simulink model "Loadflowwithsolarbasis16kWp"  (R2023a)
settings: Solver=VariableStepAuto  StartTime=0.0  StopTime=10  RelTol=1e-3
libraries: spsThreePhaseDynamicLoadLib x20, spsThreePhaseVIMeasurementLib x18, spsThreePhaseSeriesRLCBranchLib x16, spsLoadFlowBusLib x11, spsThreePhaseParallelRLCLoadLib x10, spsRMSLib x2, spsThreePhaseTransformerTwoWindingsLib x1, spsGroundLib x1, spsThreePhaseProgrammableVoltageSourceLib x1, spspowerguiLib x1
(part 1 of 2)
settings Model: Creator=KeronDenny  LastModifiedBy=KeronDenny

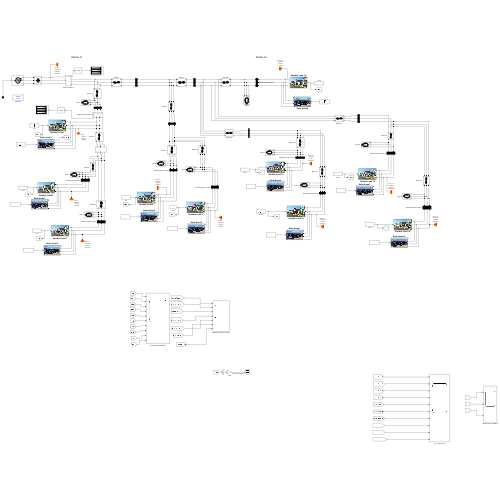
[thumbnail: Simulink's stored preview of the top-level diagram]
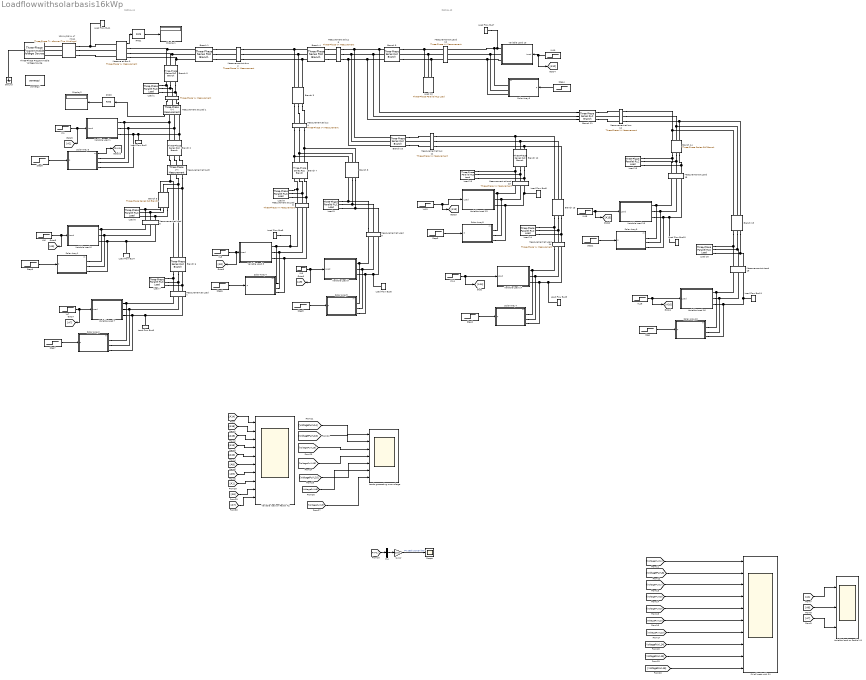
== system Loadflowwithsolarbasis16kWp ==
  note: RADIAL A1
  note: RADIAL A2
  " " : spsThreePhaseVIMeasurementLib/Three-Phase V-I Measurement  VoltageMeasurement=phase-to-ground  SetLabelV=on  LabelV=VoltagePuVL1  Vpu=on  VpuLL=off  CurrentMeasurement=no  SetLabelI=off  LabelI=Iabc  Ipu=on  Pbase=230e6  Vbase=0.230e3  OutputType=Magnitude  PhasorSimulation=on  PSBequivalent=0
  120 kV/25 kV 47 MVA1 : spsThreePhaseTransformerTwoWindingsLib/Three-Phase Transformer (Two Windings)  Winding1Connection=Yg  Winding2Connection=Yg  CoreType=Three single-phase transformers  SetSaturation=off  Hysteresis=off  DataFile='basic_model'  SetInitialFlux=off  Measurements=None  UNITS=pu  NominalPower=[230e3 50]  Winding1="[ 11e3  0.185/2/25   0.185/2 ]"  Winding2="[ 0.230e3  0.185/2/25  0.185/2]"  Rm=500  Lm=500  L0=0.5  Saturation="[ 0,0  ;  0.005,1.2  ;  1.0,1.4 ]"  InitialFluxes=[ 0.8 , -0.8 , 0.7 ]  BreakLoop=off  DiscreteSolver=Trapezoidal iterative  DataType=off  TransfoNumber=0
  Bracnh 1 : spsThreePhaseSeriesRLCBranchLib/Three-Phase Series RLC Branch  LConnTagsString=A|B|C  RConnTagsString=A|B|C  BranchType=RL  Resistance=0.216*0.240  Inductance=(0.04995*0.240)/314.159  Capacitance=1e-6  Measurements=None
  Bracnh 4 : spsThreePhaseSeriesRLCBranchLib/Three-Phase Series RLC Branch  LConnTagsString=A|B|C  RConnTagsString=A|B|C  BranchType=RL  Resistance=0.22*0.240  Inductance=(0.003*0.240)/314.159  Capacitance=1e-6  Measurements=None
  Branch 0 : spsThreePhaseSeriesRLCBranchLib/Three-Phase Series RLC Branch  LConnTagsString=A|B|C  RConnTagsString=A|B|C  BranchType=RL  Resistance=0.1824*0.240  Inductance=(0.035*0.240)/314.159  Capacitance=1e-6  Measurements=None
  Branch 10 : spsThreePhaseSeriesRLCBranchLib/Three-Phase Series RLC Branch  LConnTagsString=A|B|C  RConnTagsString=A|B|C  BranchType=RL  Resistance=0.06*0.240  Inductance=(0.004*0.240)/314.159  Capacitance=1e-6  Measurements=None
  Branch 11 : spsThreePhaseSeriesRLCBranchLib/Three-Phase Series RLC Branch  LConnTagsString=A|B|C  RConnTagsString=A|B|C  BranchType=RL  Resistance=0.032*0.240  Inductance=(0.004*0.240)/314.159  Capacitance=1e-6  Measurements=None
  Branch 12 : spsThreePhaseSeriesRLCBranchLib/Three-Phase Series RLC Branch  LConnTagsString=A|B|C  RConnTagsString=A|B|C  BranchType=RL  Resistance=0.048*0.240  Inductance=(0.003*0.240)/314.159  Capacitance=1e-6  Measurements=None
  Branch 13 : spsThreePhaseSeriesRLCBranchLib/Three-Phase Series RLC Branch  LConnTagsString=A|B|C  RConnTagsString=A|B|C  BranchType=RL  Resistance=0.042*0.240  Inductance=(0.003*0.240)/314.159  Capacitance=1e-6  Measurements=None
  Branch 14 : spsThreePhaseSeriesRLCBranchLib/Three-Phase Series RLC Branch  LConnTagsString=A|B|C  RConnTagsString=A|B|C  BranchType=RL  Resistance=0.03*0.240  Inductance=(0.002*0.240)/314.159  Capacitance=1e-6  Measurements=None
  Branch 15 : spsThreePhaseSeriesRLCBranchLib/Three-Phase Series RLC Branch  LConnTagsString=A|B|C  RConnTagsString=A|B|C  BranchType=RL  Resistance=0.042*0.240  Inductance=(0.003*0.240)/314.159  Capacitance=1e-6  Measurements=None
  Branch 2 : spsThreePhaseSeriesRLCBranchLib/Three-Phase Series RLC Branch  LConnTagsString=A|B|C  RConnTagsString=A|B|C  BranchType=RL  Resistance=0.026*0.240  Inductance=(0.003*0.240)/314.159  Capacitance=1e-6  Measurements=None
  Branch 3 : spsThreePhaseSeriesRLCBranchLib/Three-Phase Series RLC Branch  LConnTagsString=A|B|C  RConnTagsString=A|B|C  BranchType=RL  Resistance=0.06*0.240  Inductance=(0.004*0.240)/314.159  Capacitance=1e-6  Measurements=None
  Branch 5 : spsThreePhaseSeriesRLCBranchLib/Three-Phase Series RLC Branch  LConnTagsString=A|B|C  RConnTagsString=A|B|C  BranchType=RL  Resistance=0.044*0.240  Inductance=(0.003*0.240)/314.159  Capacitance=1e-6  Measurements=None
  Branch 6 : spsThreePhaseSeriesRLCBranchLib/Three-Phase Series RLC Branch  LConnTagsString=A|B|C  RConnTagsString=A|B|C  BranchType=RL  Resistance=0.023*0.240  Inductance=(0.002*0.240)/314.159  Capacitance=1e-6  Measurements=None
  Branch 7 : spsThreePhaseSeriesRLCBranchLib/Three-Phase Series RLC Branch  LConnTagsString=A|B|C  RConnTagsString=A|B|C  BranchType=RL  Resistance=0.09*0.240  Inductance=(0.006*0.240)/314.159  Capacitance=1e-6  Measurements=None
  Branch 8 : spsThreePhaseSeriesRLCBranchLib/Three-Phase Series RLC Branch  LConnTagsString=A|B|C  RConnTagsString=A|B|C  BranchType=RL  Resistance=0.072*0.240  Inductance=(0.005*0.240)/314.159  Capacitance=1e-6  Measurements=None
  Branch 9 : spsThreePhaseSeriesRLCBranchLib/Three-Phase Series RLC Branch  LConnTagsString=A|B|C  RConnTagsString=A|B|C  BranchType=RL  Resistance=0.03*0.240  Inductance=(0.002*0.240)/314.159  Capacitance=1e-6  Measurements=None
  Display1 : Display
  Display2 : Display
  Ground : spsGroundLib/Ground  LConnTagsString=a
  Load {1,6..7,13..16} (7 alike) : spsThreePhaseParallelRLCLoadLib/Three-Phase Parallel RLC Load  LConnTagsString=A|B|C  Configuration=Y (grounded)  NominalVoltage=(230)*1  Vabc=[1e3 1e3 1e3]  Vabcp=[1e3 1e3 1e3]  NominalFrequency=50  UnbalancedPower=off  ActivePower=100  InductivePower=0  CapacitivePower=2e3  Pabc=[10e3 9e3 11e3]  QLabc=[100 90 110]  QCabc=[100 90 110]  Pabcp=[10e3 9e3 11e3]  QLabcp=[100 90 110]  QCabcp=[100 90 110]  Measurements=None  LoadType=constant Z
  Load 10 : spsThreePhaseParallelRLCLoadLib/Three-Phase Parallel RLC Load  LConnTagsString=A|B|C  Configuration=Y (grounded)  NominalVoltage=(230)*1  Vabc=[1e3 1e3 1e3]  Vabcp=[1e3 1e3 1e3]  NominalFrequency=50  UnbalancedPower=off  ActivePower=100  InductivePower=0  CapacitivePower=1e3  Pabc=[10e3 9e3 11e3]  QLabc=[100 90 110]  QCabc=[100 90 110]  Pabcp=[10e3 9e3 11e3]  QLabcp=[100 90 110]  QCabcp=[100 90 110]  Measurements=None  LoadType=constant Z
  Load 8 : spsThreePhaseParallelRLCLoadLib/Three-Phase Parallel RLC Load  LConnTagsString=A|B|C  Configuration=Y (grounded)  NominalVoltage=(230)*1  Vabc=[1e3 1e3 1e3]  Vabcp=[1e3 1e3 1e3]  NominalFrequency=50  UnbalancedPower=off  ActivePower=100  InductivePower=0  CapacitivePower=1e3  Pabc=[10e3 9e3 11e3]  QLabc=[100 90 110]  QCabc=[100 90 110]  Pabcp=[10e3 9e3 11e3]  QLabcp=[100 90 110]  QCabcp=[100 90 110]  Measurements=None  LoadType=constant Z
  Load 9 : spsThreePhaseParallelRLCLoadLib/Three-Phase Parallel RLC Load  LConnTagsString=A|B|C  Configuration=Y (grounded)  NominalVoltage=(230)*1  Vabc=[1e3 1e3 1e3]  Vabcp=[1e3 1e3 1e3]  NominalFrequency=50  UnbalancedPower=off  ActivePower=100  InductivePower=0  CapacitivePower=1e3  Pabc=[10e3 9e3 11e3]  QLabc=[100 90 110]  QCabc=[100 90 110]  Pabcp=[10e3 9e3 11e3]  QLabcp=[100 90 110]  QCabcp=[100 90 110]  Measurements=None  LoadType=constant Z
  Load Flow Bus1 : spsLoadFlowBusLib/Load Flow Bus  LConnTagsString=a  Phases=single  Connectors=on one side  ID=BUS_0  Vbase=0.230e3  Vref=1  Vangle=0  VLF=0.9995  VLFb=1  VLFc=1  angleLF=3.685  angleLFb=0  angleLFc=0
  Load Flow Bus10 : spsLoadFlowBusLib/Load Flow Bus  LConnTagsString=a  Phases=single  Connectors=on one side  ID=BUS_15  Vbase=0.230e3  Vref=1  Vangle=0  VLF=1.099  VLFb=1  VLFc=1  angleLF=4.485  angleLFb=0  angleLFc=0
  Load Flow Bus11 : spsLoadFlowBusLib/Load Flow Bus  LConnTagsString=a  Phases=single  Connectors=on both sides  ID=BUS_16  Vbase=0.230e3  Vref=1  Vangle=0  VLF=1.099  VLFb=1  VLFc=1  angleLF=4.487  angleLFb=0  angleLFc=0
  Load Flow Bus2 : spsLoadFlowBusLib/Load Flow Bus  LConnTagsString=a  Phases=single  Connectors=on one side  ID=BUS_1  Vbase=0.230e3  Vref=1  Vangle=0  VLF=1.019  VLFb=1  VLFc=1  angleLF=3.896  angleLFb=0  angleLFc=0
  Load Flow Bus3 : spsLoadFlowBusLib/Load Flow Bus  LConnTagsString=a  Phases=single  Connectors=on one side  ID=BUS_7  Vbase=0.230e3  Vref=1  Vangle=0  VLF=1.021  VLFb=1  VLFc=1  angleLF=3.911  angleLFb=0  angleLFc=0
  Load Flow Bus4 : spsLoadFlowBusLib/Load Flow Bus  LConnTagsString=a  Phases=single  Connectors=on one side  ID=BUS_6  Vbase=0.230e3  Vref=1  Vangle=0  VLF=1.022  VLFb=1  VLFc=1  angleLF=3.914  angleLFb=0  angleLFc=0
  Load Flow Bus5 : spsLoadFlowBusLib/Load Flow Bus  LConnTagsString=a  Phases=single  Connectors=on one side  ID=BUS_8  Vbase=0.230e3  Vref=1  Vangle=0  VLF=1.063  VLFb=1  VLFc=1  angleLF=4.462  angleLFb=0  angleLFc=0
  Load Flow Bus6 : spsLoadFlowBusLib/Load Flow Bus  LConnTagsString=a  Phases=single  Connectors=on one side  ID=BUS_9  Vbase=0.230e3  Vref=1  Vangle=0  VLF=1.063  VLFb=1  VLFc=1  angleLF=4.46  angleLFb=0  angleLFc=0
  Load Flow Bus7 : spsLoadFlowBusLib/Load Flow Bus  LConnTagsString=a  Phases=single  Connectors=on one side  ID=BUS_10  Vbase=0.230e3  Vref=1  Vangle=0  VLF=1.097  VLFb=1  VLFc=1  angleLF=4.47  angleLFb=0  angleLFc=0
  Load Flow Bus8 : spsLoadFlowBusLib/Load Flow Bus  LConnTagsString=a  Phases=single  Connectors=on one side  ID=BUS_13  Vbase=0.230e3  Vref=1  Vangle=0  VLF=1.102  VLFb=1  VLFc=1  angleLF=4.489  angleLFb=0  angleLFc=0
  Load Flow Bus9 : spsLoadFlowBusLib/Load Flow Bus  LConnTagsString=a  Phases=single  Connectors=on one side  ID=BUS_14  Vbase=0.230e3  Vref=1  Vangle=0  VLF=1.102  VLFb=1  VLFc=1  angleLF=4.489  angleLFb=0  angleLFc=0
  Loads gnereating overvoltage : Scope  NumInputPorts=7
  Measure at Bus 0 : spsThreePhaseVIMeasurementLib/Three-Phase V-I Measurement  VoltageMeasurement=phase-to-ground  SetLabelV=off  LabelV=Vabc  Vpu=on  VpuLL=off  CurrentMeasurement=no  SetLabelI=off  LabelI=Iabc  Ipu=off  Pbase=100e6  Vbase=0.230e3  OutputType=Magnitude  PhasorSimulation=on  PSBequivalent=0
  Measurement at Laod 10 : spsThreePhaseVIMeasurementLib/Three-Phase V-I Measurement  VoltageMeasurement=phase-to-ground  SetLabelV=on  LabelV=VoltagePuVL10  Vpu=on  VpuLL=off  CurrentMeasurement=no  SetLabelI=off  LabelI=Iabc  Ipu=off  Pbase=100e6  Vbase=0.230e3  OutputType=Magnitude  PhasorSimulation=on  PSBequivalent=0
  Measurement at Laod 13 : spsThreePhaseVIMeasurementLib/Three-Phase V-I Measurement  VoltageMeasurement=phase-to-ground  SetLabelV=on  LabelV=VoltagePuVL13  Vpu=on  VpuLL=off  CurrentMeasurement=no  SetLabelI=off  LabelI=Iabc  Ipu=off  Pbase=100e6  Vbase=0.230e3  OutputType=Magnitude  PhasorSimulation=on  PSBequivalent=0
  Measurement at Load 1 : spsThreePhaseVIMeasurementLib/Three-Phase V-I Measurement  VoltageMeasurement=phase-to-ground  SetLabelV=off  LabelV=Vabc  Vpu=on  VpuLL=off  CurrentMeasurement=no  SetLabelI=off  LabelI=Iabc  Ipu=off  Pbase=100e6  Vbase=0.230e3  OutputType=Magnitude  PhasorSimulation=on  PSBequivalent=0
  Measurement at Load 14 : spsThreePhaseVIMeasurementLib/Three-Phase V-I Measurement  VoltageMeasurement=phase-to-ground  SetLabelV=on  LabelV=VoltagePuVL14  Vpu=on  VpuLL=off  CurrentMeasurement=no  SetLabelI=off  LabelI=Iabc  Ipu=off  Pbase=100e6  Vbase=0.230e3  OutputType=Magnitude  PhasorSimulation=on  PSBequivalent=0
  Measurement at Load 15 : spsThreePhaseVIMeasurementLib/Three-Phase V-I Measurement  VoltageMeasurement=phase-to-ground  SetLabelV=on  LabelV=VoltagePuVL15  Vpu=on  VpuLL=off  CurrentMeasurement=no  SetLabelI=off  LabelI=Iabc  Ipu=off  Pbase=100e6  Vbase=0.230e3  OutputType=Magnitude  PhasorSimulation=on  PSBequivalent=0
  Measurement at Load 16 : spsThreePhaseVIMeasurementLib/Three-Phase V-I Measurement  VoltageMeasurement=phase-to-ground  SetLabelV=on  LabelV=VoltagePuVL16  Vpu=on  VpuLL=off  CurrentMeasurement=no  SetLabelI=off  LabelI=Iabc  Ipu=off  Pbase=100e6  Vbase=0.230e3  OutputType=Magnitude  PhasorSimulation=on  PSBequivalent=0
  Measurement at Load 7 : spsThreePhaseVIMeasurementLib/Three-Phase V-I Measurement  VoltageMeasurement=phase-to-ground  SetLabelV=on  LabelV=VoltagePuVL7  Vpu=on  VpuLL=off  CurrentMeasurement=no  SetLabelI=off  LabelI=Iabc  Ipu=off  Pbase=100e6  Vbase=0.230e3  OutputType=Magnitude  PhasorSimulation=on  PSBequivalent=0
  Measurement at Load 8 : spsThreePhaseVIMeasurementLib/Three-Phase V-I Measurement  VoltageMeasurement=phase-to-ground  SetLabelV=on  LabelV=VoltagePuVL8  Vpu=on  VpuLL=off  CurrentMeasurement=no  SetLabelI=off  LabelI=Iabc  Ipu=off  Pbase=100e6  Vbase=0.230e3  OutputType=Magnitude  PhasorSimulation=on  PSBequivalent=0
  Measurement at Load 9 : spsThreePhaseVIMeasurementLib/Three-Phase V-I Measurement  VoltageMeasurement=phase-to-ground  SetLabelV=on  LabelV=VoltagePuVL9  Vpu=on  VpuLL=off  CurrentMeasurement=no  SetLabelI=off  LabelI=Iabc  Ipu=off  Pbase=100e6  Vbase=0.230e3  OutputType=Magnitude  PhasorSimulation=on  PSBequivalent=0
  Measurement at bus {4..5,11..12} (4 alike) : spsThreePhaseVIMeasurementLib/Three-Phase V-I Measurement  VoltageMeasurement=no  SetLabelV=off  LabelV=Vabc  Vpu=off  VpuLL=off  CurrentMeasurement=no  SetLabelI=off  LabelI=Iabc  Ipu=off  Pbase=100e6  Vbase=0.235e3  OutputType=Magnitude  PhasorSimulation=on  PSBequivalent=0
  Measurement at bus 2 : spsThreePhaseVIMeasurementLib/Three-Phase V-I Measurement  VoltageMeasurement=no  SetLabelV=off  LabelV=Vabc  Vpu=on  VpuLL=off  CurrentMeasurement=no  SetLabelI=off  LabelI=Iabc  Ipu=off  Pbase=100e6  Vbase=0.230e3  OutputType=Magnitude  PhasorSimulation=on  PSBequivalent=0
  Measurement at bus3 : spsThreePhaseVIMeasurementLib/Three-Phase V-I Measurement  VoltageMeasurement=no  SetLabelV=off  LabelV=Vabc  Vpu=off  VpuLL=on  CurrentMeasurement=no  SetLabelI=off  LabelI=Iabc  Ipu=off  Pbase=100e6  Vbase=0.230e3  OutputType=Magnitude  PhasorSimulation=on  PSBequivalent=0
  Measurement at load 6 : spsThreePhaseVIMeasurementLib/Three-Phase V-I Measurement  VoltageMeasurement=phase-to-ground  SetLabelV=on  LabelV=VoltagePuVL6  Vpu=on  VpuLL=off  CurrentMeasurement=no  SetLabelI=off  LabelI=Iabc  Ipu=off  Pbase=100e6  Vbase=0.230e3  OutputType=Magnitude  PhasorSimulation=on  PSBequivalent=0
  Mux : Mux  Inputs=1
  PU of loads with PV : Scope  NumInputPorts=10
  RMS1 : spsRMSLib/RMS  TrueRMS=on  Freq=50  RMSInit=0  Ts=0
  RMS3 : spsRMSLib/RMS  TrueRMS=on  Freq=50  RMSInit=0  Ts=0
  Scope : Scope
  Solar Array1 : Subsystem  mask(Grid-Connected PV Array (PQ Model)){Vn=230, Fn=50, P0=2000}
      mask prompts: Vn "Nominal L-L Voltage [Vrms]"; Fn "Nominal Frequency [Hz]"; P0 "Initial Power [W]"
      mask help:
      | This block models a grid-connected solar array using the Three-Phase Dynamic Load block. This is a system-level model that does not contain any power electronics, but is useful for load flow, phasor, and hybrid phasor-EMT simulations. The input to this block is the power output of the grid connected PV array, not irradiance.
      |
      | For more detailed PV models, consider the PV Array block in the Renewables library. Consider using this PQ Model to perform load flow studies and switch to a more detailed model when full EMT studies are required.
      |
      | Note: The array power must be specified for use for Load Flow analysis.
      mask init:
      | % P0 = Irr0*TotalArea*Efficiency/100;
      | P0 = -P0;
      mask Display:
      | image(imread('PV_Farm.jpg'))
      | color('white')
      | port_label('input',1,'P')
      | port_label('output',1,'m')
      | port_label('Rconn',1,'A')
      | port_label('Rconn',2,'B')
      | port_label('Rconn',3,'C')
  Solar Array10 : Subsystem  mask(Grid-Connected PV Array (PQ Model)){Vn=230, Fn=50, P0=2000}
      mask prompts: Vn "Nominal L-L Voltage [Vrms]"; Fn "Nominal Frequency [Hz]"; P0 "Initial Power [W]"
      mask help:
      | This block models a grid-connected solar array using the Three-Phase Dynamic Load block. This is a system-level model that does not contain any power electronics, but is useful for load flow, phasor, and hybrid phasor-EMT simulations. The input to this block is the power output of the grid connected PV array, not irradiance.
      |
      | For more detailed PV models, consider the PV Array block in the Renewables library. Consider using this PQ Model to perform load flow studies and switch to a more detailed model when full EMT studies are required.
      |
      | Note: The array power must be specified for use for Load Flow analysis.
      mask init:
      | % P0 = Irr0*TotalArea*Efficiency/100;
      | P0 = -P0;
      mask Display:
      | image(imread('PV_Farm.jpg'))
      | color('white')
      | port_label('input',1,'P')
      | port_label('output',1,'m')
      | port_label('Rconn',1,'A')
      | port_label('Rconn',2,'B')
      | port_label('Rconn',3,'C')
  Solar Array2 : Subsystem  mask(Grid-Connected PV Array (PQ Model)){Vn=230, Fn=50, P0=2000}
      mask prompts: Vn "Nominal L-L Voltage [Vrms]"; Fn "Nominal Frequency [Hz]"; P0 "Initial Power [W]"
      mask help:
      | This block models a grid-connected solar array using the Three-Phase Dynamic Load block. This is a system-level model that does not contain any power electronics, but is useful for load flow, phasor, and hybrid phasor-EMT simulations. The input to this block is the power output of the grid connected PV array, not irradiance.
      |
      | For more detailed PV models, consider the PV Array block in the Renewables library. Consider using this PQ Model to perform load flow studies and switch to a more detailed model when full EMT studies are required.
      |
      | Note: The array power must be specified for use for Load Flow analysis.
      mask init:
      | % P0 = Irr0*TotalArea*Efficiency/100;
      | P0 = -P0;
      mask Display:
      | image(imread('PV_Farm.jpg'))
      | color('white')
      | port_label('input',1,'P')
      | port_label('output',1,'m')
      | port_label('Rconn',1,'A')
      | port_label('Rconn',2,'B')
      | port_label('Rconn',3,'C')
  Solar Array3 : Subsystem  mask(Grid-Connected PV Array (PQ Model)){Vn=230, Fn=50, P0=2000}
      mask prompts: Vn "Nominal L-L Voltage [Vrms]"; Fn "Nominal Frequency [Hz]"; P0 "Initial Power [W]"
      mask help:
      | This block models a grid-connected solar array using the Three-Phase Dynamic Load block. This is a system-level model that does not contain any power electronics, but is useful for load flow, phasor, and hybrid phasor-EMT simulations. The input to this block is the power output of the grid connected PV array, not irradiance.
      |
      | For more detailed PV models, consider the PV Array block in the Renewables library. Consider using this PQ Model to perform load flow studies and switch to a more detailed model when full EMT studies are required.
      |
      | Note: The array power must be specified for use for Load Flow analysis.
      mask init:
      | % P0 = Irr0*TotalArea*Efficiency/100;
      | P0 = -P0;
      mask Display:
      | image(imread('PV_Farm.jpg'))
      | color('white')
      | port_label('input',1,'P')
      | port_label('output',1,'m')
      | port_label('Rconn',1,'A')
      | port_label('Rconn',2,'B')
      | port_label('Rconn',3,'C')
  Solar Array4 : Subsystem  mask(Grid-Connected PV Array (PQ Model)){Vn=230, Fn=50, P0=2000}
      mask prompts: Vn "Nominal L-L Voltage [Vrms]"; Fn "Nominal Frequency [Hz]"; P0 "Initial Power [W]"
      mask help:
      | This block models a grid-connected solar array using the Three-Phase Dynamic Load block. This is a system-level model that does not contain any power electronics, but is useful for load flow, phasor, and hybrid phasor-EMT simulations. The input to this block is the power output of the grid connected PV array, not irradiance.
      |
      | For more detailed PV models, consider the PV Array block in the Renewables library. Consider using this PQ Model to perform load flow studies and switch to a more detailed model when full EMT studies are required.
      |
      | Note: The array power must be specified for use for Load Flow analysis.
      mask init:
      | % P0 = Irr0*TotalArea*Efficiency/100;
      | P0 = -P0;
      mask Display:
      | image(imread('PV_Farm.jpg'))
      | color('white')
      | port_label('input',1,'P')
      | port_label('output',1,'m')
      | port_label('Rconn',1,'A')
      | port_label('Rconn',2,'B')
      | port_label('Rconn',3,'C')
  Solar Array5 : Subsystem  mask(Grid-Connected PV Array (PQ Model)){Vn=230, Fn=50, P0=2000}
      mask prompts: Vn "Nominal L-L Voltage [Vrms]"; Fn "Nominal Frequency [Hz]"; P0 "Initial Power [W]"
      mask help:
      | This block models a grid-connected solar array using the Three-Phase Dynamic Load block. This is a system-level model that does not contain any power electronics, but is useful for load flow, phasor, and hybrid phasor-EMT simulations. The input to this block is the power output of the grid connected PV array, not irradiance.
      |
      | For more detailed PV models, consider the PV Array block in the Renewables library. Consider using this PQ Model to perform load flow studies and switch to a more detailed model when full EMT studies are required.
      |
      | Note: The array power must be specified for use for Load Flow analysis.
      mask init:
      | % P0 = Irr0*TotalArea*Efficiency/100;
      | P0 = -P0;
      mask Display:
      | image(imread('PV_Farm.jpg'))
      | color('white')
      | port_label('input',1,'P')
      | port_label('output',1,'m')
      | port_label('Rconn',1,'A')
      | port_label('Rconn',2,'B')
      | port_label('Rconn',3,'C')
  Solar Array6 : Subsystem  mask(Grid-Connected PV Array (PQ Model)){Vn=230, Fn=50, P0=2000}
      mask prompts: Vn "Nominal L-L Voltage [Vrms]"; Fn "Nominal Frequency [Hz]"; P0 "Initial Power [W]"
      mask help:
      | This block models a grid-connected solar array using the Three-Phase Dynamic Load block. This is a system-level model that does not contain any power electronics, but is useful for load flow, phasor, and hybrid phasor-EMT simulations. The input to this block is the power output of the grid connected PV array, not irradiance.
      |
      | For more detailed PV models, consider the PV Array block in the Renewables library. Consider using this PQ Model to perform load flow studies and switch to a more detailed model when full EMT studies are required.
      |
      | Note: The array power must be specified for use for Load Flow analysis.
      mask init:
      | % P0 = Irr0*TotalArea*Efficiency/100;
      | P0 = -P0;
      mask Display:
      | image(imread('PV_Farm.jpg'))
      | color('white')
      | port_label('input',1,'P')
      | port_label('output',1,'m')
      | port_label('Rconn',1,'A')
      | port_label('Rconn',2,'B')
      | port_label('Rconn',3,'C')
  Solar Array7 : Subsystem  mask(Grid-Connected PV Array (PQ Model)){Vn=230, Fn=50, P0=2000}
      mask prompts: Vn "Nominal L-L Voltage [Vrms]"; Fn "Nominal Frequency [Hz]"; P0 "Initial Power [W]"
      mask help:
      | This block models a grid-connected solar array using the Three-Phase Dynamic Load block. This is a system-level model that does not contain any power electronics, but is useful for load flow, phasor, and hybrid phasor-EMT simulations. The input to this block is the power output of the grid connected PV array, not irradiance.
      |
      | For more detailed PV models, consider the PV Array block in the Renewables library. Consider using this PQ Model to perform load flow studies and switch to a more detailed model when full EMT studies are required.
      |
      | Note: The array power must be specified for use for Load Flow analysis.
      mask init:
      | % P0 = Irr0*TotalArea*Efficiency/100;
      | P0 = -P0;
      mask Display:
      | image(imread('PV_Farm.jpg'))
      | color('white')
      | port_label('input',1,'P')
      | port_label('output',1,'m')
      | port_label('Rconn',1,'A')
      | port_label('Rconn',2,'B')
      | port_label('Rconn',3,'C')
  Solar Array8 : Subsystem  mask(Grid-Connected PV Array (PQ Model)){Vn=230, Fn=50, P0=2000}
      mask prompts: Vn "Nominal L-L Voltage [Vrms]"; Fn "Nominal Frequency [Hz]"; P0 "Initial Power [W]"
      mask help:
      | This block models a grid-connected solar array using the Three-Phase Dynamic Load block. This is a system-level model that does not contain any power electronics, but is useful for load flow, phasor, and hybrid phasor-EMT simulations. The input to this block is the power output of the grid connected PV array, not irradiance.
      |
      | For more detailed PV models, consider the PV Array block in the Renewables library. Consider using this PQ Model to perform load flow studies and switch to a more detailed model when full EMT studies are required.
      |
      | Note: The array power must be specified for use for Load Flow analysis.
      mask init:
      | % P0 = Irr0*TotalArea*Efficiency/100;
      | P0 = -P0;
      mask Display:
      | image(imread('PV_Farm.jpg'))
      | color('white')
      | port_label('input',1,'P')
      | port_label('output',1,'m')
      | port_label('Rconn',1,'A')
      | port_label('Rconn',2,'B')
      | port_label('Rconn',3,'C')
  Solar Array9 : Subsystem  mask(Grid-Connected PV Array (PQ Model)){Vn=230, Fn=50, P0=2000}
      mask prompts: Vn "Nominal L-L Voltage [Vrms]"; Fn "Nominal Frequency [Hz]"; P0 "Initial Power [W]"
      mask help:
      | This block models a grid-connected solar array using the Three-Phase Dynamic Load block. This is a system-level model that does not contain any power electronics, but is useful for load flow, phasor, and hybrid phasor-EMT simulations. The input to this block is the power output of the grid connected PV array, not irradiance.
      |
      | For more detailed PV models, consider the PV Array block in the Renewables library. Consider using this PQ Model to perform load flow studies and switch to a more detailed model when full EMT studies are required.
      |
      | Note: The array power must be specified for use for Load Flow analysis.
      mask init:
      | % P0 = Irr0*TotalArea*Efficiency/100;
      | P0 = -P0;
      mask Display:
      | image(imread('PV_Farm.jpg'))
      | color('white')
      | port_label('input',1,'P')
      | port_label('output',1,'m')
      | port_label('Rconn',1,'A')
      | port_label('Rconn',2,'B')
      | port_label('Rconn',3,'C')
  Step{,1..9} (10 alike) : Step  Time=5  Before=2000  After=16300  SampleTime=0
  Three-Phase Programmable Voltage Source : spsThreePhaseProgrammableVoltageSourceLib/Three-Phase Programmable Voltage Source  PositiveSequence=[(11000)*1 0 50]  VariationEntity=None  VariationType=Modulation  VariationTypeAlt=Step  VariationStep=0.5  VariationRate=0.1  VariationMagnitude=0.05  VariationFrequency=1  VariationTiming=[0.1 1.2]  VariationPhaseA=off  Amplitudes=[1 0.8 1.2 1.0]  TimeValues=[0 0.1 0.15 0.2]  HarmonicGeneration=off  HarmonicA=[3 0.2 -25 0]  HarmonicB=[2 0.15 35 2]  Timing="[0.05  3]"  BusType=swing  Pref=0  Qref=0  Qmin=-Inf  Qmax=Inf
  VL1 : Step  Time=1.5  Before=1e2  After=6.119e3  SampleTime=0
  VL10 : Step  Time=0.2  Before=1e2  After=5.191e3  SampleTime=0
  VL13 : Step  Time=0.6  Before=2e2  After=7.979e3  SampleTime=0
  VL14 : Step  Before=9e2  After=5.457e3  SampleTime=0
  VL15 : Step  Time=0.1  Before=6e2  After=5.473e3  SampleTime=0
  VL16 : Step  Time=0.5  Before=10  After=5.191e3  SampleTime=0
  VL6 : Step  Time=0.9  Before=4e2  After=2.018e3  SampleTime=0
  VL7 : Step  Time=0.3  Before=8e2  After=5.178e3  SampleTime=0
  VL8 : Step  Time=0.5  Before=1e2  After=6.662e3  SampleTime=0
  VL9 : Step  Time=1.5  Before=1e2  After=3.414e3  SampleTime=0
  Variable Load 1 : Subsystem  mask(Variable Load (PQ Model)){Vn=230, Fn=50, PF=1, Load0=1e2}
      mask prompts: Vn "Nominal L-L Voltage [Vrms]"; Fn "Nominal Frequency [Hz]"; PF "Power Factor [0 to 1]"; Load0 "Initial Load [W]"
      mask help:
      | The Variable Load block is a lumped approximation for a distribution feeder. For non-unity power factor loads, the input (active power) is scaled accordingly to generate a desired load.
      |
      | Note: The initial input load must be specified for use for Load Flow analysis.
      mask init:
      | P0 = Load0;
      | Q0 = Load0*sqrt(1/PF-1);
      mask Display:
      | image(imread('Residential.jpg'))
      | color('white')
      | port_label('input',1,'Load')
      | port_label('Rconn',1,'A')
      | port_label('Rconn',2,'B')
      | port_label('Rconn',3,'C')
  Variable Load 10 : Subsystem  mask(Variable Load (PQ Model)){Vn=230, Fn=50, PF=1, Load0=1e2}
      mask prompts: Vn "Nominal L-L Voltage [Vrms]"; Fn "Nominal Frequency [Hz]"; PF "Power Factor [0 to 1]"; Load0 "Initial Load [W]"
      mask help:
      | The Variable Load block is a lumped approximation for a distribution feeder. For non-unity power factor loads, the input (active power) is scaled accordingly to generate a desired load.
      |
      | Note: The initial input load must be specified for use for Load Flow analysis.
      mask init:
      | P0 = Load0;
      | Q0 = Load0*sqrt(1/PF-1);
      mask Display:
      | image(imread('Residential.jpg'))
      | color('white')
      | port_label('input',1,'Load')
      | port_label('Rconn',1,'A')
      | port_label('Rconn',2,'B')
      | port_label('Rconn',3,'C')
  Variable Load 13 : Subsystem  mask(Variable Load (PQ Model)){Vn=230, Fn=50, PF=1, Load0=1e2}
      mask prompts: Vn "Nominal L-L Voltage [Vrms]"; Fn "Nominal Frequency [Hz]"; PF "Power Factor [0 to 1]"; Load0 "Initial Load [W]"
      mask help:
      | The Variable Load block is a lumped approximation for a distribution feeder. For non-unity power factor loads, the input (active power) is scaled accordingly to generate a desired load.
      |
      | Note: The initial input load must be specified for use for Load Flow analysis.
      mask init:
      | P0 = Load0;
      | Q0 = Load0*sqrt(1/PF-1);
      mask Display:
      | image(imread('Residential.jpg'))
      | color('white')
      | port_label('input',1,'Load')
      | port_label('Rconn',1,'A')
      | port_label('Rconn',2,'B')
      | port_label('Rconn',3,'C')
  Variable Load 14 : Subsystem  mask(Variable Load (PQ Model)){Vn=230, Fn=50, PF=1, Load0=1e2}
      mask prompts: Vn "Nominal L-L Voltage [Vrms]"; Fn "Nominal Frequency [Hz]"; PF "Power Factor [0 to 1]"; Load0 "Initial Load [W]"
      mask help:
      | The Variable Load block is a lumped approximation for a distribution feeder. For non-unity power factor loads, the input (active power) is scaled accordingly to generate a desired load.
      |
      | Note: The initial input load must be specified for use for Load Flow analysis.
      mask init:
      | P0 = Load0;
      | Q0 = Load0*sqrt(1/PF-1);
      mask Display:
      | image(imread('Residential.jpg'))
      | color('white')
      | port_label('input',1,'Load')
      | port_label('Rconn',1,'A')
      | port_label('Rconn',2,'B')
      | port_label('Rconn',3,'C')
  Variable Load 15 : Subsystem  mask(Variable Load (PQ Model)){Vn=230, Fn=50, PF=1, Load0=1e2}
      mask prompts: Vn "Nominal L-L Voltage [Vrms]"; Fn "Nominal Frequency [Hz]"; PF "Power Factor [0 to 1]"; Load0 "Initial Load [W]"
      mask help:
      | The Variable Load block is a lumped approximation for a distribution feeder. For non-unity power factor loads, the input (active power) is scaled accordingly to generate a desired load.
      |
      | Note: The initial input load must be specified for use for Load Flow analysis.
      mask init:
      | P0 = Load0;
      | Q0 = Load0*sqrt(1/PF-1);
      mask Display:
      | image(imread('Residential.jpg'))
      | color('white')
      | port_label('input',1,'Load')
      | port_label('Rconn',1,'A')
      | port_label('Rconn',2,'B')
      | port_label('Rconn',3,'C')
  Variable Load 16 : Subsystem  mask(Variable Load (PQ Model)){Vn=230, Fn=50, PF=1, Load0=1e2}
      mask prompts: Vn "Nominal L-L Voltage [Vrms]"; Fn "Nominal Frequency [Hz]"; PF "Power Factor [0 to 1]"; Load0 "Initial Load [W]"
      mask help:
      | The Variable Load block is a lumped approximation for a distribution feeder. For non-unity power factor loads, the input (active power) is scaled accordingly to generate a desired load.
      |
      | Note: The initial input load must be specified for use for Load Flow analysis.
      mask init:
      | P0 = Load0;
      | Q0 = Load0*sqrt(1/PF-1);
      mask Display:
      | image(imread('Residential.jpg'))
      | color('white')
      | port_label('input',1,'Load')
      | port_label('Rconn',1,'A')
      | port_label('Rconn',2,'B')
      | port_label('Rconn',3,'C')
  Variable Load 6 : Subsystem  mask(Variable Load (PQ Model)){Vn=230, Fn=50, PF=1, Load0=7500}
      mask prompts: Vn "Nominal L-L Voltage [Vrms]"; Fn "Nominal Frequency [Hz]"; PF "Power Factor [0 to 1]"; Load0 "Initial Load [W]"
      mask help:
      | The Variable Load block is a lumped approximation for a distribution feeder. For non-unity power factor loads, the input (active power) is scaled accordingly to generate a desired load.
      |
      | Note: The initial input load must be specified for use for Load Flow analysis.
      mask init:
      | P0 = Load0;
      | Q0 = Load0*sqrt(1/PF-1);
      mask Display:
      | image(imread('Residential.jpg'))
      | color('white')
      | port_label('input',1,'Load')
      | port_label('Rconn',1,'A')
      | port_label('Rconn',2,'B')
      | port_label('Rconn',3,'C')
  Variable Load 7 : Subsystem  mask(Variable Load (PQ Model)){Vn=230, Fn=50, PF=1, Load0=1e2}
      mask prompts: Vn "Nominal L-L Voltage [Vrms]"; Fn "Nominal Frequency [Hz]"; PF "Power Factor [0 to 1]"; Load0 "Initial Load [W]"
      mask help:
      | The Variable Load block is a lumped approximation for a distribution feeder. For non-unity power factor loads, the input (active power) is scaled accordingly to generate a desired load.
      |
      | Note: The initial input load must be specified for use for Load Flow analysis.
      mask init:
      | P0 = Load0;
      | Q0 = Load0*sqrt(1/PF-1);
      mask Display:
      | image(imread('Residential.jpg'))
      | color('white')
      | port_label('input',1,'Load')
      | port_label('Rconn',1,'A')
      | port_label('Rconn',2,'B')
      | port_label('Rconn',3,'C')
  Variable Load 8 : Subsystem  mask(Variable Load (PQ Model)){Vn=230, Fn=50, PF=1, Load0=1e2}
      mask prompts: Vn "Nominal L-L Voltage [Vrms]"; Fn "Nominal Frequency [Hz]"; PF "Power Factor [0 to 1]"; Load0 "Initial Load [W]"
      mask help:
      | The Variable Load block is a lumped approximation for a distribution feeder. For non-unity power factor loads, the input (active power) is scaled accordingly to generate a desired load.
      |
      | Note: The initial input load must be specified for use for Load Flow analysis.
      mask init:
      | P0 = Load0;
      | Q0 = Load0*sqrt(1/PF-1);
      mask Display:
      | image(imread('Residential.jpg'))
      | color('white')
      | port_label('input',1,'Load')
      | port_label('Rconn',1,'A')
      | port_label('Rconn',2,'B')
      | port_label('Rconn',3,'C')
  Variable Load 9 : Subsystem  mask(Variable Load (PQ Model)){Vn=230, Fn=50, PF=1, Load0=1e2}
      mask prompts: Vn "Nominal L-L Voltage [Vrms]"; Fn "Nominal Frequency [Hz]"; PF "Power Factor [0 to 1]"; Load0 "Initial Load [W]"
      mask help:
      | The Variable Load block is a lumped approximation for a distribution feeder. For non-unity power factor loads, the input (active power) is scaled accordingly to generate a desired load.
      |
      | Note: The initial input load must be specified for use for Load Flow analysis.
      mask init:
      | P0 = Load0;
      | Q0 = Load0*sqrt(1/PF-1);
      mask Display:
      | image(imread('Residential.jpg'))
      | color('white')
      | port_label('input',1,'Load')
      | port_label('Rconn',1,'A')
      | port_label('Rconn',2,'B')
      | port_label('Rconn',3,'C')
  Variable load on Radial A1 : Scope  NumInputPorts=3
  Variable load on Radial A2 : Scope  NumInputPorts=10
  powergui : spspowerguiLib/powergui  Priority=1  SimulationMode=Phasor  SampleTime=50e-6  frequency=50  Iterations=50  frequencyindice=50  Pbase=100e3  ErrMax=1e-4  UnitsV=kV  UnitsW=MW  buscounter=0  FunctionMessages=off  echomessages=off  EnableUseOfTLC=off  CurrentSourceSwitches=off  DisableSnubberDevices=off  DisableRonSwitches=off  DisableVfSwitches=off  DisplayEquations=off  AutomaticDiscreteSolvers=off  SolverType=Tustin/Backward Euler (TBE)  Interpol=off  ExternalGateDelay=off  methode=off  Ts=100  x0status=blocks  SPID=on  SwTol=0  HookPort=off  NonlinearTolerance=1e-4  nMaxIteration=100  ContinueOnMaxIteration=off  RestoreLinks=warning  ResistiveCurrentMeasurement=off  Frange=[0:2:500]  Ylog=off  Xlog=on  ShowGrid=off  save=off  variable=ZData  structure=0  ZoomFFT=off  StartTime=0.0  cycles=1  DisplayStyle=1  fundamental=60  FreqAxis=off  MaxFrequency=1000  frequencyindicesteady=1  RmsSteady=1  display=off
  to kW : Gain  Gain=1e-3
  wires:
  Measure at Bus 0/1 -> RMS1/1
  RMS1/1 -> Display1/1
  Measurement at Load 1/1 -> RMS3/1
  RMS3/1 -> Display2/1
  VL6/1 -> [A6], Variable Load 6/1(Load)
  VL1/1 -> [A1], Variable Load 1/1(Load)
  VL7/1 -> [A7], Variable Load 7/1(Load)
  VL8/1 -> [A8], Variable Load 8/1(Load)
  VL9/1 -> [A9], Variable Load 9/1(Load)
  VL15/1 -> Variable Load 15/1(Load), [A15]
  VL16/1 -> Variable Load 16/1(Load), [A16]
  VL14/1 -> Variable Load 14/1(Load), [A14]
  [A14] -> Variable load on Radial A2/1
  [A16] -> Variable load on Radial A2/2
  [A15] -> Variable load on Radial A2/3
  VL13/1 -> Variable Load 13/1(Load), [A13]
  [A13] -> Variable load on Radial A2/4
  VL10/1 -> [A10], Variable Load 10/1(Load)
  [A10] -> Variable load on Radial A2/5
  [A9] -> Variable load on Radial A2/7
  [A8] -> Variable load on Radial A2/6
  [A1] -> Variable load on Radial A1/1
  [A6] -> Variable load on Radial A1/2
  [A7] -> Variable load on Radial A1/3
  Solar Array3/1(m) -> [PVM1]
  Mux/1 -> to kW/1
  to kW/1 -> Scope/1  "PV peak power (kW)"
  [PVM1] -> Mux/1
  Step4/1 -> Solar Array6/1(P)
  Step/1 -> Solar Array10/1(P)
  Step1/1 -> Solar Array9/1(P)
  [VoltagePuVL6] -> PU of loads with PV/2
  [VoltagePuVL1] -> PU of loads with PV/1
  [VoltagePuVL7] -> PU of loads with PV/3
  [VoltagePuVL8] -> PU of loads with PV/4
  [VoltagePuVL9] -> PU of loads with PV/5
  [VoltagePuVL10] -> PU of loads with PV/6
  [VoltagePuVL13] -> PU of loads with PV/7
  [VoltagePuVL14] -> PU of loads with PV/8
  [VoltagePuVL15] -> PU of loads with PV/9
  [VoltagePuVL16] -> PU of loads with PV/10
  [VoltagePuVL14] -> Loads gnereating overvoltage/1
  [VoltagePuVL13] -> Loads gnereating overvoltage/2
  [VoltagePuVL16] -> Loads gnereating overvoltage/3
  [VoltagePuVL15] -> Loads gnereating overvoltage/4
  Step2/1 -> Solar Array7/1(P)
  Step3/1 -> Solar Array8/1(P)
  Step5/1 -> Solar Array5/1(P)
  Step6/1 -> Solar Array4/1(P)
  Step7/1 -> Solar Array2/1(P)
  Step9/1 -> Solar Array1/1(P)
  [VoltagePuVL10] -> Loads gnereating overvoltage/5
  Step8/1 -> Solar Array3/1(P)
  [VoltagePuVL8] -> Loads gnereating overvoltage/6
  [VoltagePuVL9] -> Loads gnereating overvoltage/7
  [A1] -> Variable load on Radial A2/8
  [A6] -> Variable load on Radial A2/9
  [A7] -> Variable load on Radial A2/10
  connections:
  Branch 0/RConn3 -- Load 1/LConn3 -- " "/LConn3
  Branch 0/RConn2 -- Load 1/LConn2 -- " "/LConn2
  Branch 0/RConn1 -- " "/LConn1 -- Load 1/LConn1
  Measurement at Load 1/LConn1 -- " "/RConn1
  Measurement at Load 1/LConn2 -- " "/RConn2
  Measurement at Load 1/LConn3 -- " "/RConn3
  Three-Phase Programmable Voltage Source/LConn1 -- Ground/LConn1
  Branch 2/LConn1 -- Solar Array3/RConn1 -- Variable Load 1/RConn1 -- Measurement at Load 1/RConn1
  Branch 2/LConn2 -- Solar Array3/RConn2 -- Variable Load 1/RConn2 -- Measurement at Load 1/RConn2
  Measurement at Load 1/RConn3 -- Solar Array3/RConn3 -- Variable Load 1/RConn3 -- Load Flow Bus2/LConn1 -- Branch 2/LConn3
  Measure at Bus 0/RConn1 -- Bracnh 1/LConn1 -- Branch 0/LConn1
  Measure at Bus 0/RConn2 -- Bracnh 1/LConn2 -- Branch 0/LConn2
  Measure at Bus 0/RConn3 -- Bracnh 1/LConn3 -- Branch 0/LConn3
  Bracnh 1/RConn1 -- Measurement at bus 2/LConn1
  Bracnh 1/RConn2 -- Measurement at bus 2/LConn2
  Bracnh 1/RConn3 -- Measurement at bus 2/LConn3
  Branch 2/RConn1 -- Measurement at bus3/LConn1
  Branch 2/RConn2 -- Measurement at bus3/LConn2
  Branch 2/RConn3 -- Measurement at bus3/LConn3
  Measurement at bus 2/RConn1 -- Branch 3/LConn1 -- Bracnh 4/LConn1
  Measurement at bus 2/RConn2 -- Branch 3/LConn2 -- Bracnh 4/LConn2
  Measurement at bus 2/RConn3 -- Branch 3/LConn3 -- Bracnh 4/LConn3
  Branch 3/RConn1 -- Measurement at bus 4/LConn1
  Branch 3/RConn2 -- Measurement at bus 4/LConn2
  Branch 3/RConn3 -- Measurement at bus 4/LConn3
  Measurement at bus 5/LConn2 -- Bracnh 4/RConn2
  Bracnh 4/RConn3 -- Measurement at bus 5/LConn3
  Bracnh 4/RConn1 -- Measurement at bus 5/LConn1
  Branch 5/LConn1 -- Branch 6/LConn1 -- Measurement at bus3/RConn1
  Branch 6/LConn2 -- Branch 5/LConn2 -- Measurement at bus3/RConn2
  Measurement at bus3/RConn3 -- Branch 5/LConn3 -- Branch 6/LConn3
  Branch 5/RConn1 -- Measurement at load 6/LConn1 -- Load 6/LConn1
  Branch 5/RConn2 -- Measurement at load 6/LConn2 -- Load 6/LConn2
  Branch 5/RConn3 -- Measurement at load 6/LConn3 -- Load 6/LConn3
  Measurement at Load 7/LConn3 -- Load 7/LConn3 -- Branch 6/RConn3
  Branch 6/RConn2 -- Load 7/LConn2 -- Measurement at Load 7/LConn2
  Branch 6/RConn1 -- Load 7/LConn1 -- Measurement at Load 7/LConn1
  Measurement at bus 4/RConn1 -- Branch 7/LConn1 -- Branch 8/LConn1
  Measurement at bus 4/RConn2 -- Branch 7/LConn2 -- Branch 8/LConn2
  Measurement at bus 4/RConn3 -- Branch 7/LConn3 -- Branch 8/LConn3
  Load 8/LConn1 -- Measurement at Load 8/LConn1 -- Branch 7/RConn1
  Branch 7/RConn2 -- Load 8/LConn2 -- Measurement at Load 8/LConn2
  Branch 7/RConn3 -- Load 8/LConn3 -- Measurement at Load 8/LConn3
  Measurement at Load 9/LConn1 -- Branch 8/RConn1 -- Load 9/LConn1
  Branch 8/RConn2 -- Load 9/LConn2 -- Measurement at Load 9/LConn2
  Branch 8/RConn3 -- Load 9/LConn3 -- Measurement at Load 9/LConn3
  Measurement at bus 5/RConn1 -- Branch 10/LConn1 -- Branch 11/LConn1 -- Branch 9/LConn1
  Measurement at bus 5/RConn2 -- Branch 10/LConn2 -- Branch 11/LConn2 -- Branch 9/LConn2
  Measurement at bus 5/RConn3 -- Branch 10/LConn3 -- Branch 11/LConn3 -- Branch 9/LConn3
  Measurement at Laod 10/LConn2 -- Load 10/LConn2 -- Branch 9/RConn2
  Branch 9/RConn3 -- Load 10/LConn3 -- Measurement at Laod 10/LConn3
  Branch 9/RConn1 -- Load 10/LConn1 -- Measurement at Laod 10/LConn1
  Measurement at bus 11/LConn2 -- Branch 10/RConn2
  Branch 10/RConn1 -- Measurement at bus 11/LConn1
  Branch 10/RConn3 -- Measurement at bus 11/LConn3
  Branch 11/RConn3 -- Measurement at bus 12/LConn3
  Branch 11/RConn1 -- Measurement at bus 12/LConn1
  Measurement at bus 12/LConn2 -- Branch 11/RConn2
  Measurement at bus 11/RConn1 -- Branch 13/LConn1 -- Branch 12/LConn1
  Measurement at bus 11/RConn2 -- Branch 13/LConn2 -- Branch 12/LConn2
  Measurement at bus 11/RConn3 -- Branch 13/LConn3 -- Branch 12/LConn3
  Branch 12/RConn1 -- Measurement at Laod 13/LConn1 -- Load 13/LConn1
  Branch 12/RConn2 -- Load 13/LConn2 -- Measurement at Laod 13/LConn2
  Branch 12/RConn3 -- Load 13/LConn3 -- Measurement at Laod 13/LConn3
  Load 14/LConn1 -- Measurement at Load 14/LConn1 -- Branch 13/RConn1
  Branch 13/RConn2 -- Measurement at Load 14/LConn2 -- Load 14/LConn2
  Load 14/LConn3 -- Measurement at Load 14/LConn3 -- Branch 13/RConn3
  Branch 14/RConn1 -- Measurement at Load 15/LConn1 -- Load 15/LConn1
  Branch 14/RConn2 -- Load 15/LConn2 -- Measurement at Load 15/LConn2
  Branch 14/RConn3 -- Measurement at Load 15/LConn3 -- Load 15/LConn3
  Load 16/LConn1 -- Measurement at Load 16/LConn1 -- Branch 15/RConn1
  Branch 15/RConn2 -- Measurement at Load 16/LConn2 -- Load 16/LConn2
  Load 16/LConn3 -- Measurement at Load 16/LConn3 -- Branch 15/RConn3
  Measurement at bus 12/RConn1 -- Branch 15/LConn1 -- Branch 14/LConn1
  Measurement at bus 12/RConn2 -- Branch 15/LConn2 -- Branch 14/LConn2
  Measurement at bus 12/RConn3 -- Branch 15/LConn3 -- Branch 14/LConn3
  Measurement at load 6/RConn1 -- Solar Array1/RConn1 -- Variable Load 6/RConn1
  Variable Load 6/RConn2 -- Solar Array1/RConn2 -- Measurement at load 6/RConn2
  Variable Load 6/RConn3 -- Solar Array1/RConn3 -- Measurement at load 6/RConn3 -- Load Flow Bus4/LConn1
  Variable Load 7/RConn1 -- Solar Array2/RConn1 -- Measurement at Load 7/RConn1
  Variable Load 7/RConn2 -- Solar Array2/RConn2 -- Measurement at Load 7/RConn2
  Variable Load 7/RConn3 -- Solar Array2/RConn3 -- Load Flow Bus3/LConn1 -- Measurement at Load 7/RConn3
  Variable Load 8/RConn1 -- Solar Array4/RConn1 -- Load Flow Bus5/LConn1 -- Measurement at Load 8/RConn1
  Variable Load 8/RConn2 -- Solar Array4/RConn2 -- Measurement at Load 8/RConn2
  Variable Load 10/RConn2 -- Solar Array6/RConn2 -- Measurement at Laod 10/RConn2
  Variable Load 10/RConn1 -- Load Flow Bus7/LConn1 -- Solar Array6/RConn1 -- Measurement at Laod 10/RConn1
  Variable Load 15/RConn1 -- Solar Array9/RConn1 -- Measurement at Load 15/RConn1
  Variable Load 15/RConn2 -- Solar Array9/RConn2 -- Measurement at Load 15/RConn2
  Variable Load 15/RConn3 -- Measurement at Load 15/RConn3 -- Load Flow Bus10/LConn1 -- Solar Array9/RConn3
  Variable Load 16/RConn1 -- Solar Array10/RConn1 -- Measurement at Load 16/RConn1
  Variable Load 16/RConn2 -- Solar Array10/RConn2 -- Measurement at Load 16/RConn2
  Variable Load 16/RConn3 -- Solar Array10/RConn3 -- Load Flow Bus11/LConn1 -- Measurement at Load 16/RConn3
  Variable Load 13/RConn1 -- Solar Array8/RConn1 -- Measurement at Laod 13/RConn1
  Variable Load 13/RConn2 -- Solar Array8/RConn2 -- Measurement at Laod 13/RConn2
  Variable Load 13/RConn3 -- Solar Array8/RConn3 -- Load Flow Bus8/LConn1 -- Measurement at Laod 13/RConn3
  Variable Load 14/RConn3 -- Solar Array7/RConn3 -- Load Flow Bus9/LConn1 -- Measurement at Load 14/RConn3
  Variable Load 14/RConn2 -- Solar Array7/RConn2 -- Measurement at Load 14/RConn2
  Measurement at Load 14/RConn1 -- Solar Array7/RConn1 -- Variable Load 14/RConn1
  Variable Load 8/RConn3 -- Solar Array4/RConn3 -- Measurement at Load 8/RConn3
  Variable Load 9/RConn1 -- Measurement at Load 9/RConn1 -- Solar Array5/RConn1
  Variable Load 9/RConn2 -- Solar Array5/RConn2 -- Measurement at Load 9/RConn2
  Variable Load 9/RConn3 -- Solar Array5/RConn3 -- Measurement at Load 9/RConn3 -- Load Flow Bus6/LConn1
  Variable Load 10/RConn3 -- Solar Array6/RConn3 -- Measurement at Laod 10/RConn3
  120 kV/25 kV 47 MVA1/LConn1 -- Three-Phase Programmable Voltage Source/RConn1
  120 kV/25 kV 47 MVA1/LConn2 -- Three-Phase Programmable Voltage Source/RConn2
  120 kV/25 kV 47 MVA1/LConn3 -- Three-Phase Programmable Voltage Source/RConn3
  120 kV/25 kV 47 MVA1/RConn1 -- Load Flow Bus1/LConn1 -- Measure at Bus 0/LConn1
  120 kV/25 kV 47 MVA1/RConn2 -- Measure at Bus 0/LConn2
  120 kV/25 kV 47 MVA1/RConn3 -- Measure at Bus 0/LConn3

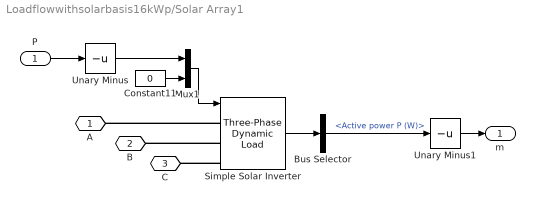
== system Loadflowwithsolarbasis16kWp/Solar Array1 ==
  P : Inport
  Bus Selector : BusSelector  OutputSignals=Active power P (W)
  Constant11 : Constant  Value=0
  Mux1 : Mux  Inputs=2
  Simple Solar Inverter : spsThreePhaseDynamicLoadLib/Three-Phase Dynamic Load  NominalVoltage=[Vn Fn]  ActiveReactivePowers=[-16300 -3.38813e-13]  PositiveSequence=[1.0994 4.48658]  ExternalControl=on  NpNq=[1.3 2]  TimeConstants="[0  0  0  0]"  MinimumVoltage=0.7  Tfilter=1e-2  LoadFlowParameters=[4,0,0,0,0]
      settings: LibrarySourceBlock=|
      | sps_lib/Passives/Three-Phase
      | Dynamic Load
  Unary Minus : UnaryMinus
  Unary Minus1 : UnaryMinus
  A : PMIOPort  Side=Right
  B : PMIOPort  Port=2  Side=Right
  C : PMIOPort  Port=3  Side=Right
  m : Outport  VectorParamsAs1DForOutWhenUnconnected=off
  wires:
  Unary Minus1/1 -> m/1
  Bus Selector/1 -> Unary Minus1/1  "<Active power P (W)>"
  Simple Solar Inverter/1 -> Bus Selector/1
  Constant11/1 -> Mux1/2
  Mux1/1 -> Simple Solar Inverter/1
  Unary Minus/1 -> Mux1/1
  P/1 -> Unary Minus/1
  connections:
  Simple Solar Inverter/LConn1 -- A/RConn1
  Simple Solar Inverter/LConn3 -- C/RConn1
  Simple Solar Inverter/LConn2 -- B/RConn1

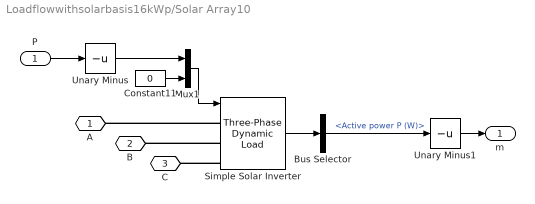
== system Loadflowwithsolarbasis16kWp/Solar Array10 ==
  P : Inport
  Bus Selector : BusSelector  OutputSignals=Active power P (W)
  Constant11 : Constant  Value=0
  Mux1 : Mux  Inputs=2
  Simple Solar Inverter : spsThreePhaseDynamicLoadLib/Three-Phase Dynamic Load  NominalVoltage=[Vn Fn]  ActiveReactivePowers=[-15000 -3.38813e-13]  PositiveSequence=[1.0994 4.48658]  ExternalControl=on  NpNq=[1.3 2]  TimeConstants="[0  0  0  0]"  MinimumVoltage=0.7  Tfilter=1e-2  LoadFlowParameters=[4,0,0,0,0]
      settings: LibrarySourceBlock=|
      | sps_lib/Passives/Three-Phase
      | Dynamic Load
  Unary Minus : UnaryMinus
  Unary Minus1 : UnaryMinus
  A : PMIOPort  Side=Right
  B : PMIOPort  Port=2  Side=Right
  C : PMIOPort  Port=3  Side=Right
  m : Outport  VectorParamsAs1DForOutWhenUnconnected=off
  wires:
  P/1 -> Unary Minus/1
  Unary Minus/1 -> Mux1/1
  Mux1/1 -> Simple Solar Inverter/1
  Constant11/1 -> Mux1/2
  Simple Solar Inverter/1 -> Bus Selector/1
  Bus Selector/1 -> Unary Minus1/1  "<Active power P (W)>"
  Unary Minus1/1 -> m/1
  connections:
  Simple Solar Inverter/LConn2 -- B/RConn1
  Simple Solar Inverter/LConn3 -- C/RConn1
  Simple Solar Inverter/LConn1 -- A/RConn1

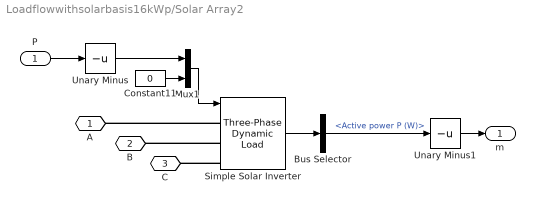
== system Loadflowwithsolarbasis16kWp/Solar Array2 ==
  P : Inport
  Bus Selector : BusSelector  OutputSignals=Active power P (W)
  Constant11 : Constant  Value=0
  Mux1 : Mux  Inputs=2
  Simple Solar Inverter : spsThreePhaseDynamicLoadLib/Three-Phase Dynamic Load  NominalVoltage=[Vn Fn]  ActiveReactivePowers=[-16300 -3.38813e-13]  PositiveSequence=[1.0994 4.48658]  ExternalControl=on  NpNq=[1.3 2]  TimeConstants="[0  0  0  0]"  MinimumVoltage=0.7  Tfilter=1e-2  LoadFlowParameters=[4,0,0,0,0]
      settings: LibrarySourceBlock=|
      | sps_lib/Passives/Three-Phase
      | Dynamic Load
  Unary Minus : UnaryMinus
  Unary Minus1 : UnaryMinus
  A : PMIOPort  Side=Right
  B : PMIOPort  Port=2  Side=Right
  C : PMIOPort  Port=3  Side=Right
  m : Outport  VectorParamsAs1DForOutWhenUnconnected=off
  wires:
  P/1 -> Unary Minus/1
  Unary Minus/1 -> Mux1/1
  Mux1/1 -> Simple Solar Inverter/1
  Constant11/1 -> Mux1/2
  Simple Solar Inverter/1 -> Bus Selector/1
  Bus Selector/1 -> Unary Minus1/1  "<Active power P (W)>"
  Unary Minus1/1 -> m/1
  connections:
  Simple Solar Inverter/LConn2 -- B/RConn1
  Simple Solar Inverter/LConn3 -- C/RConn1
  Simple Solar Inverter/LConn1 -- A/RConn1
